simulink model "Tutorial_Simulink_6"  (R2023b)
settings: Solver=VariableStepAuto  StartTime=0.0  StopTime=10.0  RelTol=1e-3
model workspace (MAT data in the model file):
  F = 0
  b = Simulink.Parameter
  b.Value = 0.6
  b.DataType = 'auto'
  b.Complexity = 'real'
  b.Dimensions = [1 1]
  k = 5
  m = 1
  v0 = 0
  x0 = 10
settings Model: Creator=admin  LastModifiedBy=admin

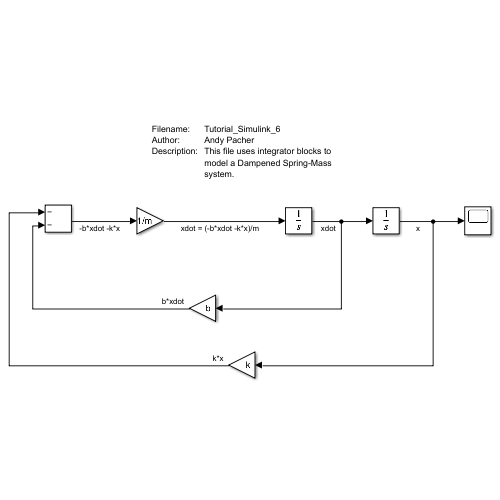
[thumbnail: Simulink's stored preview of the top-level diagram]
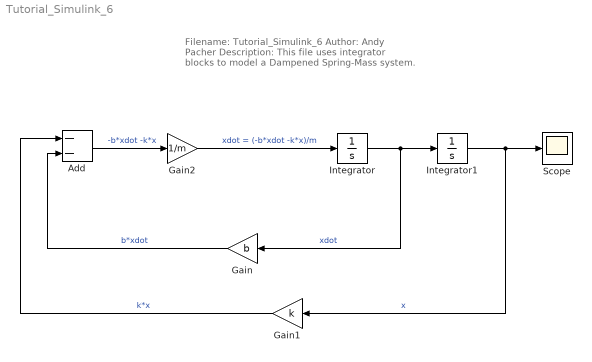
== system Tutorial_Simulink_6 ==
  note: Filename:	Tutorial_Simulink_6
      | Author:		Andy Pacher
      | Description:	This file uses integrator blocks to
      | 			model a Dampened Spring-Mass
      | 			system.
  Add : Sum  Inputs=--
  Gain : Gain  Gain=b
  Gain1 : Gain  Gain=k
  Gain2 : Gain  Gain=1/m
  Integrator : Integrator
  Integrator1 : Integrator  InitialCondition=x0
  Scope : Scope
  wires:
  Gain2/1 -> Integrator/1  "xdot = (-b*xdot -k*x)/m"
  Integrator1/1 -> Gain1/1, Scope/1  "x"
  Integrator/1 -> Gain/1, Integrator1/1  "xdot"
  Gain1/1 -> Add/1  "k*x"
  Gain/1 -> Add/2  "b*xdot"
  Add/1 -> Gain2/1  "-b*xdot -k*x"
